simulink model "article"  (R2020a)
settings: Solver=FixedStepAuto  StartTime=0.0  StopTime=5  FixedStep=2e-4  RelTol=1e-3  AbsTol=1e-3
libraries: fl_lib x8, nesl_utility x7, ee_lib x2
settings Model: OrderedModelArguments=off  Creator=Anzin  LastModifiedBy=Anzin
settings OptimizationCC: OptimizeBlockIOStorage=off  BufferReuse=off  OptimizeDataStoreBuffers=off  BusAssignmentInplaceUpdate=off
settings DebuggingCC: SignalInfNanChecking=error  SFUnexpectedBacktrackingDiag=warning  SFNoUnconditionalDefaultTransitionDiag=warning
settings HardwareCC: ProdHWDeviceType=AMD->x86-64 (Windows64)
settings RTWCC: GenerateReport=on  BuildConfiguration=Debug  LaunchReport=on
settings CodeAppCC: ForceParamTrailComments=on  MATLABSourceComments=on  EnableCustomComments=on
settings GRTTargetCC: CombineSignalStateStructs=on  SupportVariableSizeSignals=on  MultiInstanceErrorCode=Warning

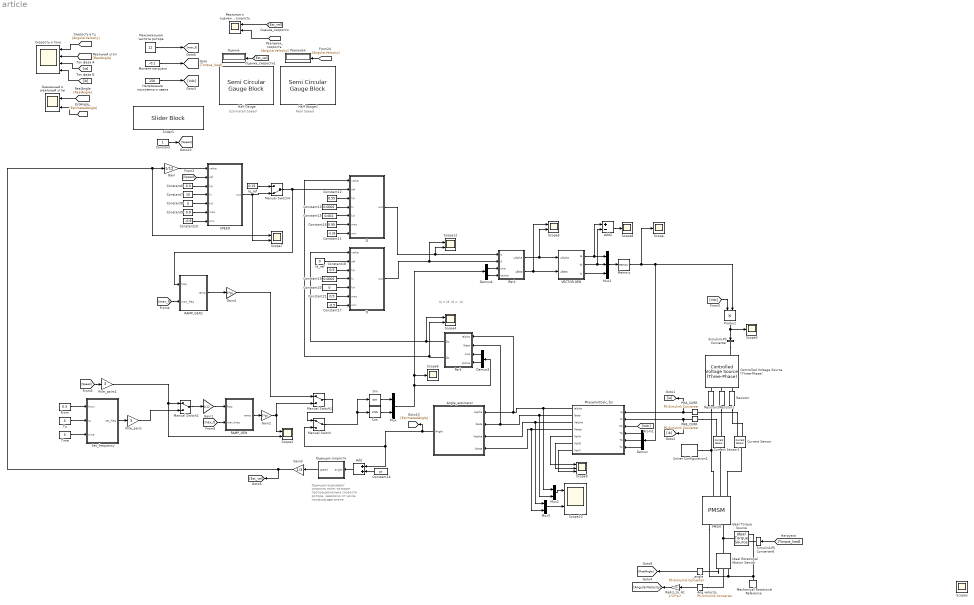
== system article ==
  note: Оценщик оценивает скорость поля, которая пропорциональна скорости ротора, зависимо от числа полюсов двигателя
  note: Real Speed
  note: Estimated Speed
  note: Iq = Id'
      | Id = -Iq'
  Add : Sum
  Add2 : Sum  Inputs=+-
  Ang velocity : nesl_utility/PS-Simulink Converter  PhysicalDomain=network_engine_domain  SubClassName=ps_output  LeftPortType=input  RightPortType=output  PseudoPeriodic=off  Frequencies=[]  Unit=inherit  AffineConversion=off
  Angle_estimator : MATLAB Function  TreatAsAtomicUnit=on
  Constant : Constant
  Constant10 : Constant  Value=-0.9
  Constant11 : Constant  Value=-0.95
  Constant12 : Constant  Value=0.55
  Constant13 : Constant  Value=0.0002
  Constant14 : Constant  Value=pi
  Constant15 : Constant  Value=0.001
  Constant16 : Constant  Value=0.95
  Constant17 : Constant  Value=-0.5
  Constant18 : Constant  Value=0.5
  Constant19 : Constant  Value=0.0002
  Constant20 : Constant  Value=0
  Constant21 : Constant  Value=0.5
  Constant6 : Constant  Value=0.3
  Constant7 : Constant  Value=10
  Constant8 : Constant  Value=0
  Constant9 : Constant  Value=0.9
  Controlled Voltage Source (Three-Phase) : ee_lib/Sources/Controlled Voltage Source (Three-Phase)
      settings: SourceProductBaseCode=PS  InternalSimscapePortConfiguration="{\"Bottom\":[],\"Left\":[{\"id\":\"S\",\"label\":\"S\",\"type\":\"input\"},{\"id\":\"n\",\"label\":\"n\",\"type\":\"foundation.electrical.electrical\"}],\"Right\":[{\"id\":\"a\",\"label\":\"a\",\"type\":\"foundation.electrical.electrical\"},{\"id\":\"b\",\"label\":\"b\",\"type\":\"foundation.electrical.electrical\"},{\"id\":\"c\",\"label\":\"c\",\"type\":\"foundation.electrical.electrical\"}],\"Top\":[]}"
  Cos : Trigonometry  Operator=cos
  Current Sensor : fl_lib/Electrical/Electrical Sensors/Current Sensor
      settings: SourceProductBaseCode=MT,SS
  Current Sensor1 : fl_lib/Electrical/Electrical Sensors/Current Sensor
      settings: SourceProductBaseCode=MT,SS
  D : MATLAB Function  TreatAsAtomicUnit=on
  Demux : Demux  Outputs=3
  Demux3 : Demux  Outputs=2
  Demux4 : Demux  Outputs=2
  From : Constant  Value=0.3
  Gain : Gain  Gain=1/12
  Gain1 : Gain  Gain=1/12
  Gain2 : Gain  Gain=2*pi
  Gain3 : Gain  Gain=1/3
  Gain4 : Gain  Gain=2*pi
  Half Gauge : SemiCircularGaugeBlock  ScaleMin=-12  ScaleMax=12
  Half Gauge1 : SemiCircularGaugeBlock  ScaleMin=-12  ScaleMax=12
  IPark : MATLAB Function  TreatAsAtomicUnit=on
  Id_ref : Constant  Value=0
  Ideal Rotational Motion Sensor : fl_lib/Mechanical/Mechanical Sensors/Ideal Rotational Motion Sensor  wrap_angle=simscape.enum.onoff.on  offset=0 rad
  Ideal Torque Source : fl_lib/Mechanical/Mechanical Sources/Ideal Torque Source
  Iq_ref : Constant  Value=0.15
  Manual Switch : ManualSwitch
  Manual Switch1 : ManualSwitch
  Manual Switch2 : ManualSwitch
  Manual Switch4 : ManualSwitch  CurrentSetting=0
  Mechanical Rotational Reference : fl_lib/Mechanical/Rotational Elements/Mechanical Rotational Reference
  Memory : Memory
  Mux : Mux  Inputs=2
  Mux1 : Mux  Inputs=3
  Mux2 : Mux  Inputs=2
  Mux3 : Mux  Inputs=2
  PHA_CURR : nesl_utility/PS-Simulink Converter  PhysicalDomain=network_engine_domain  SubClassName=ps_output  LeftPortType=input  RightPortType=output  PseudoPeriodic=off  Frequencies=[]  Unit=inherit  AffineConversion=off
  PHB_CURR : nesl_utility/PS-Simulink Converter  PhysicalDomain=network_engine_domain  SubClassName=ps_output  LeftPortType=input  RightPortType=output  PseudoPeriodic=off  Frequencies=[]  Unit=inherit  AffineConversion=off
  PMSM : ee_lib/Electromechanical/Permanent Magnet/PMSM  winding_type=ee.enum.statorconnection.wye  machine_param=ee.enum.pmsm.parameterization.constant  nPolePairs=3  pmflux_param=ee.enum.pmflux.backemfconstant  pm_flux_linkage=0.03 Wb  torque_constant=0.18 N*m/A  back_emf_constant=0.147 V/rpm  stator_param=ee.enum.statorparam.LdLqL0  Ld=10 mH  Lq=5 mH  idVec=[-200, 0, 200] A  iqVec=[-200, 0, 200] A  LdMatrix=0.0002 * ones(3, 3) H  LqMatrix=0.0002 * ones(3, 3) H  PmMatrix=0.1 * ones(3, 3) Wb  ktMatrix=0.18 * ones(3, 3) N*m/A  keMatrix=0.18 * ones(3, 3) V/(rad/s)  L0=7.5 mH  Ls=0.0002 H  Lm=-0.00002 H  Ms=0.00002 H  Rs=0.31 Ohm  zero_sequence=ee.enum.park.zerosequence.include  J=214e-4 kg*m^2  lam=0 N*m/(rad/s)  axes_param=ee.enum.rotorangle.daxis  i_d_specify=off  i_d_priority=None  i_d=0 A  i_d_nominal_specify=off  i_d_nominal_unit=A  i_d_nominal_value=1  i_q_specify=off  i_q_priority=None  i_q=0 A  i_q_nominal_specify=off  i_q_nominal_unit=A  i_q_nominal_value=1  torque_specify=off  torque_priority=None  torque=0 N*m  torque_nominal_specify=off  torque_nominal_unit=N*m  torque_nominal_value=1  angular_velocity_specify=off  angular_velocity_priority=High  angular_velocity=450 rpm  angular_velocity_nominal_specify=off  angular_velocity_nominal_unit=rpm  angular_velocity_nominal_value=1  angular_position_specify=off  angular_position_priority=High  angular_position=30 deg  angular_position_nominal_specify=off  angular_position_nominal_unit=deg  angular_position_nominal_value=1  loss_param=ee.enum.ironloss.none  losses_oc=[0, 0, 0] W  losses_sc=[0, 0, 0] W  f_losses=60 Hz  Isc_losses=95 A  Tmeas=298.15 K  alpha=3.93e-3 1/K  alpha_flux=-0.001 1/K  stator_thermal_mass=100 J/K  rotor_thermal_mass=200 J/K  Rm_percent_rotor=90  Rd_percent_rotor=30  temperatureA_specify=off  temperatureA_priority=High  temperatureA=25 degC  temperatureA_nominal_specify=off  temperatureA_nominal_unit=degC  temperatureA_nominal_value=1  temperatureB_specify=off  temperatureB_priority=High  temperatureB=25 degC  temperatureB_nominal_specify=off  temperatureB_nominal_unit=degC  temperatureB_nominal_value=1  temperatureC_specify=off  temperatureC_priority=High  temperatureC=25 degC  temperatureC_nominal_specify=off  temperatureC_nominal_unit=degC  temperatureC_nominal_value=1  temperatureR_specify=off  temperatureR_priority=High  temperatureR=25 degC  temperatureR_nominal_specify=off  temperatureR_nominal_unit=degC  temperatureR_nominal_value=1
      settings: InternalSimscapePortConfiguration="{\"Bottom\":[],\"Left\":[{\"id\":\"a\",\"label\":\"a\",\"type\":\"foundation.electrical.electrical\"},{\"id\":\"b\",\"label\":\"b\",\"type\":\"foundation.electrical.electrical\"},{\"id\":\"c\",\"label\":\"c\",\"type\":\"foundation.electrical.electrical\"},{\"id\":\"n\",\"label\":\"n\",\"type\":\"foundation.electrical.electrical\"}],\"Right\":[{\"id\":\"R\",\"label\":\"R\",\"type\":\"foundation.mechanical.rotational.rotational\"},{\"id\":\"C\",\"label\":\"C\",\"type\":\"foundation.mechanical.rotational.rotational\"}],\"Top\":[]}"
  Park : MATLAB Function  TreatAsAtomicUnit=on
  PhaseVoltCalc_fcn : MATLAB Function  TreatAsAtomicUnit=on
  Pole_pairs : Gain  Gain=3
  Pole_pairs1 : Gain  Gain=3
  Product : Product
  Q : MATLAB Function  TreatAsAtomicUnit=on
  RAMP_GEN : MATLAB Function  TreatAsAtomicUnit=on
  RAMP_GEN1 : MATLAB Function  TreatAsAtomicUnit=on
  Rad/s_to_Hz : Gain  Gain=1/(2*pi)
  Resistor : fl_lib/Electrical/Electrical Elements/Resistor  R=2 Ohm  i_specify=off  i_priority=None  i=0 A  i_nominal_specify=off  i_nominal_unit=A  i_nominal_value=1  v_specify=off  v_priority=None  v=0 V  v_nominal_specify=off  v_nominal_unit=V  v_nominal_value=1
  Resistor1 : fl_lib/Electrical/Electrical Elements/Resistor  R=2 Ohm  i_specify=off  i_priority=None  i=0 A  i_nominal_specify=off  i_nominal_unit=A  i_nominal_value=1  v_specify=off  v_priority=None  v=0 V  v_nominal_specify=off  v_nominal_unit=V  v_nominal_value=1
  Resistor2 : fl_lib/Electrical/Electrical Elements/Resistor  R=2 Ohm  i_specify=off  i_priority=None  i=0 A  i_nominal_specify=off  i_nominal_unit=A  i_nominal_value=1  v_specify=off  v_priority=None  v=0 V  v_nominal_specify=off  v_nominal_unit=V  v_nominal_value=1
  SPEED : MATLAB Function  TreatAsAtomicUnit=on
  Scope{,1,3,6,8} (5 alike) : Scope
  Scope{2,4..5,7,10,12} (6 alike) : Scope  NumInputPorts=2
  Scope9 : Scope  NumInputPorts=3
  Set_frequency : MATLAB Function  TreatAsAtomicUnit=on
  Simulink-PS Converter : nesl_utility/Simulink-PS Converter  PhysicalDomain=network_engine_domain  SubClassName=ps_input  LeftPortType=input  RightPortType=output  PseudoPeriodic=off  Frequencies=[]  NoiseDistribution=none  NoiseParameters=[]  Unit=1  AffineConversion=off  FilteringAndDerivatives=provide  SimscapeFilterOrder=1  InputFilterTimeConstant=0.001  UdotUserProvided=0
  Simulink-PS Converter6 : nesl_utility/Simulink-PS Converter  PhysicalDomain=network_engine_domain  SubClassName=ps_input  LeftPortType=input  RightPortType=output  PseudoPeriodic=off  Frequencies=[]  NoiseDistribution=none  NoiseParameters=[]  Unit=1  AffineConversion=off  FilteringAndDerivatives=provide  SimscapeFilterOrder=1  InputFilterTimeConstant=0.001  UdotUserProvided=0
  Sin : Trigonometry
  Slider1 : SliderBlock  ScaleMax=12
  Solver Configuration1 : nesl_utility/Solver Configuration  PhysicalDomain=network_engine_domain  SubClassName=solver  LeftPortType=input  RightPortType=generic  Tones=[]  Harmonics=[]  SimulateNoise=off  Profile=off  UseLocalSampling=off  EnableSwitchedLinearOptims=on  FrequencyDomain=off  UseCCode=off  RelTol=0.001  AbsTol=1e-06  MinStep=1e-09  ToWorkspace=off  RevertToSquareIcSolve=off  NumHomotopyIterations=100  PhasorMode=off  PhasorModeNumHarmonics=1  DoDC=off  ResidualTolerance=1e-09  UseLocalSolver=off  LocalSolverChoice=NE_BACKWARD_EULER_ADVANCER  LocalSolverSampleTime=0.001  DoFixedCost=off  MaxNonlinIter=3  MaxModeIter=2  LinearAlgebra=auto  EquationFormulation=NE_TIME_EF  DelaysMemoryBudget=1024  AutomaticFiltering=on  FilteringTimeConstant=0.001  PartitionStorageMethod=AS_NEEDED  PartitionMemoryBudget=1024  PartitionMethod=ROBUST
  Time : Constant  Value=5
  To : Constant  Value=5
  VECTOR GEN : MATLAB Function  TreatAsAtomicUnit=on
  _angle : nesl_utility/PS-Simulink Converter  PhysicalDomain=network_engine_domain  SubClassName=ps_output  LeftPortType=input  RightPortType=output  PseudoPeriodic=off  Frequencies=[]  Unit=inherit  AffineConversion=off
  Максимальная частота ротора : Constant  Value=12
  Момент нагрузки : Constant  Value=-0.1
  Напряжение постоянного звена : Constant  Value=150  SampleTime=-1
  Оцененный и реальный углы : Scope  NumInputPorts=2
  Оценка : Display
      settings: Decimation=3
  Оценщик скорости : MATLAB Function  TreatAsAtomicUnit=on
  Реальная : Display
      settings: Decimation=3
  Реальная и оцененная скорость : Scope  NumInputPorts=2
  Скорость и токи : Scope  NumInputPorts=4
  wires:
  Момент нагрузки/1 -> [Torque_load]
  Напряжение постоянного звена/1 -> [Vdc]
  Time/1 -> Set_frequency/3(time)
  [Torque_load] -> Simulink-PS Converter6/1
  [RealAngle] -> Скорость и токи/2
  [AngularVelocity] -> Скорость и токи/1
  [ia] -> Скорость и токи/3
  [ib] -> Скорость и токи/4
  [EstimatedAngle] -> Оцененный и реальный углы/2
  [Est_vel] -> Оценка/1
  [AngularVelocity] -> Реальная/1
  From/1 -> Set_frequency/1(from)
  To/1 -> Set_frequency/2(to)
  [Est_vel] -> Реальная и оцененная скорость/1
  [AngularVelocity] -> Реальная и оцененная скорость/2
  [Speed] -> Pole_pairs1/1
  Add/1 -> Оценщик скорости/1(angle)
  IPark/2(uBeta) -> Scope5/1, VECTOR GEN/2(uBeta)
  IPark/1(uAlpha) -> Scope5/2, VECTOR GEN/1(uAlpha)
  Constant14/1 -> Add/2
  PHA_CURR/1 -> PhaseVoltCalc_fcn/1(ia), [ia]
  Ang velocity/1 -> Rad/s_to_Hz/1
  Rad/s_to_Hz/1 -> [AngularVelocity]
  _angle/1 -> [RealAngle]
  [Vdc] -> PhaseVoltCalc_fcn/3(Vd)
  Demux/1 -> PhaseVoltCalc_fcn/4(Ta)
  Demux/2 -> PhaseVoltCalc_fcn/5(Tb)
  Demux/3 -> PhaseVoltCalc_fcn/6(Tc)
  PhaseVoltCalc_fcn/1(Ialpha) -> Mux2/1, Park/1(Ialpha), Angle_estimator/1(Ialpha)
  PhaseVoltCalc_fcn/2(Ibeta) -> Mux2/2, Park/2(Ibeta), Angle_estimator/2(Ibeta)
  PhaseVoltCalc_fcn/3(Valpha) -> Mux3/1, Angle_estimator/3(Valpha)
  PhaseVoltCalc_fcn/4(Vbeta) -> Mux3/2, Angle_estimator/4(Vbeta)
  Angle_estimator/1(Angle) -> [EstimatedAngle], Add/1, Manual Switch/2
  Manual Switch/1 -> Sin/1, Cos/1
  Cos/1 -> Mux/2
  Sin/1 -> Mux/1
  [Speed] -> SPEED/2(ref)
  Constant6/1 -> SPEED/3(kp)
  Constant7/1 -> SPEED/4(ki)
  Constant8/1 -> SPEED/5(kd)
  Constant9/1 -> SPEED/6(max)
  Constant10/1 -> SPEED/7(min)
  Оценщик скорости/1(speed) -> Gain3/1
  SPEED/1(out) -> Scope7/2, Manual Switch4/2
  Iq_ref/1 -> Manual Switch4/1
  Park/1(Ds) -> D/1(value), Scope4/1
  Constant11/1 -> Q/7(min)
  Constant16/1 -> Q/6(max)
  Constant15/1 -> Q/5(kd)
  Constant13/1 -> Q/4(ki)
  Constant12/1 -> Q/3(kp)
  Constant17/1 -> D/7(min)
  Constant21/1 -> D/6(max)
  Constant20/1 -> D/5(kd)
  Constant18/1 -> D/3(kp)
  Constant19/1 -> D/4(ki)
  Id_ref/1 -> D/2(ref)
  Park/2(Qs) -> Q/1(value), Scope4/2
  VECTOR GEN/1(ta) -> Add2/1, Mux1/1
  VECTOR GEN/2(tb) -> Add2/2, Mux1/2
  VECTOR GEN/3(tc) -> Mux1/3
  Constant/1 -> [Speed]
  Mux1/1 -> Memory/1
  Memory/1 -> Scope/1, Product/2, Demux/1
  Set_frequency/1(set_freq) -> Pole_pairs/1
  Product/1 -> Scope3/1, Simulink-PS Converter/1
  [Vdc] -> Product/1
  [RealAngle] -> Оцененный и реальный углы/1
  Gain/1 -> SPEED/1(value)
  Mux/1 -> Scope6/1, Demux4/1, Demux3/1
  Demux3/1 -> Park/3(sine)
  Demux3/2 -> Park/4(cosine)
  Demux4/1 -> IPark/3(sine)
  Demux4/2 -> IPark/4(cosine)
  Pole_pairs1/1 -> Scope2/2, Manual Switch2/1
  Pole_pairs/1 -> Manual Switch2/2
  Gain1/1 -> RAMP_GEN/1(freq)
  Manual Switch2/1 -> Gain1/1
  RAMP_GEN/1(ramp) -> Gain2/1
  Gain2/1 -> Scope2/1, Manual Switch1/2
  Add2/1 -> Scope8/1
  PhaseVoltCalc_fcn/5(VphA) -> Scope9/1
  PhaseVoltCalc_fcn/6(VphB) -> Scope9/2
  PhaseVoltCalc_fcn/7(VphC) -> Scope9/3
  Mux2/1 -> Scope10/1
  Mux3/1 -> Scope10/2
  PHB_CURR/1 -> [ib], PhaseVoltCalc_fcn/2(ib)
  Gain3/1 -> [Est_vel], Scope7/1, Gain/1
  Manual Switch4/1 -> RAMP_GEN1/1(freq), Q/2(ref)
  Q/1(out) -> Scope12/2, IPark/1(q)
  D/1(out) -> Scope12/1, IPark/2(d)
  RAMP_GEN1/1(ramp) -> Gain4/1
  Manual Switch1/1 -> Manual Switch/1
  Gain4/1 -> Manual Switch1/1
  Максимальная частота ротора/1 -> [max_f]
  [max_f] -> RAMP_GEN1/2(max_freq)
  [max_f] -> RAMP_GEN/2(max_freq)
  connections:
  PHA_CURR/LConn1 -- Current Sensor/RConn1
  PHB_CURR/LConn1 -- Current Sensor1/RConn1
  Simulink-PS Converter/RConn1 -- Controlled Voltage Source (Three-Phase)/LConn1
  Ideal Rotational Motion Sensor/LConn1 -- Ideal Torque Source/LConn1 -- PMSM/RConn1
  Mechanical Rotational Reference/LConn1 -- PMSM/RConn2 -- Ideal Rotational Motion Sensor/RConn1 -- Ideal Torque Source/RConn2
  Simulink-PS Converter6/RConn1 -- Ideal Torque Source/RConn1
  Ideal Rotational Motion Sensor/RConn3 -- _angle/LConn1
  Ang velocity/LConn1 -- Ideal Rotational Motion Sensor/RConn2
  Resistor2/LConn1 -- Controlled Voltage Source (Three-Phase)/RConn3
  Resistor1/LConn1 -- Controlled Voltage Source (Three-Phase)/RConn2
  Resistor/LConn1 -- Controlled Voltage Source (Three-Phase)/RConn1
  Resistor/RConn1 -- Current Sensor/RConn2
  Resistor1/RConn1 -- Current Sensor1/RConn2
  Resistor2/RConn1 -- PMSM/LConn3 -- Solver Configuration1/RConn1
  Current Sensor1/LConn1 -- PMSM/LConn2
  PMSM/LConn1 -- Current Sensor/LConn1

== matlab function article/RAMP_GEN1 ==
  data: freq input; ramp output; max_freq input
function ramp = Ramp(freq, max_freq)

persistent angle;
persistent prevAngle;

if isempty(angle)
    angle = 0;
end

if isempty(prevAngle)
    prevAngle = 0;
end

step = freq * max_freq * 2e-4;
angle = angle + step;

if angle >= 1
    angle = angle - 1;
end

ramp = angle;

== matlab function article/Оценщик скорости ==
  data: angle input; speed output
function speed = spdest(angle)

persistent prevAngle;
persistent prevSpeed;
persistent p_speed;
persistent counter;
persistent overall;

if isempty(overall)
    overall = 0;
end

if isempty(counter)
    counter = 0;
end

if isempty(p_speed)
    p_speed = 0;
end

if isempty(prevAngle)
    prevAngle = 0;
end

if isempty(prevSpeed)
    prevSpeed = 0;
end


if angle < prevAngle
    temp = (2 * pi) - prevAngle + angle;
else
    temp = angle - prevAngle;
end

prev_speed = 0.3 * ((temp * 5000) / 6.28) + 0.7 * (prevSpeed);
overall = overall + prev_speed;
counter = counter + 1;
prevSpeed = prev_speed;
prevAngle = angle;

if counter >= 500
    speed = overall / 500;
    p_speed = speed;
    counter = 0;
    overall = 0;
else
    speed = p_speed;
end

== matlab function article/Angle_estimator ==
  settings: updateMethod=DISCRETE
  data: Ialpha input; Angle output; Ibeta input; Valpha input; Vbeta input
function Angle = AngleEstimator(Ialpha, Ibeta, Valpha, Vbeta)

persistent prevIalpha;
persistent prevIbeta;
persistent L0;
persistent L1;
persistent angle;

if isempty(prevIalpha)
    prevIalpha = 0;
end

if isempty(prevIbeta)
    prevIbeta = 0;
end

if isempty(L0)
    L0 = (5e-3 + 10e-3) / 2;
end

if isempty(L1)
    L1 = (10e-3 - 5e-3) / 2;
end

if isempty(angle)
    angle = 0;
end

Ealpha = Valpha - 0.31 * Ialpha - (L0 + L1 * cos(2 * angle)) * (Ialpha - prevIalpha) / 2e-4;
Ebeta = Vbeta - 0.31 * Ibeta - (L0 - L1 * cos(2 * angle)) * (Ibeta - prevIbeta) / 2e-4;
prevIalpha = Ialpha;
prevIbeta = Ibeta;
Angle = atan2(-Ealpha, Ebeta);
angle = Angle;

== matlab function article/IPark ==
  data: q input; d input; uAlpha output; sine input; uBeta output; cosine input
function [uAlpha, uBeta]= IPark(q, d, sine, cosine)

%преобразование увеличивает амплитуду на 2/sqrt(3), делю обратно

% uAlpha = (d * cosine - q * sine) / (2 / sqrt(3));
% uBeta = (q * cosine + d * sine) / (2 / sqrt(3));

uAlpha = d * cosine - q * sine;
uBeta = q * cosine + d * sine;

== matlab function article/VECTOR GEN ==
  data: uAlpha input size=1; ta output size=1; uBeta input size=1; tb output size=1; tc output size=1
function [ta, tb, tc] = svgen(uAlpha, uBeta)

%здесь делают обратное преобразование кларк, но оно не такое как в книге
%калачева, если что взять оттуда и проверить
%попробовать код оттуда'

tmp1 = uBeta;
tmp2 = uBeta * 0.5 + uAlpha * (sqrt(3) / 2);
tmp3 = tmp2 - tmp1;

sector = 3;
if tmp2 > 0
    sector = sector - 1;
end

if tmp3 > 0
    sector = sector - 1;
end

if tmp1 < 0
    sector = 7 - sector;
end

if sector == 1 || sector == 4
    ta = tmp2; %значения прериодов нужно снормировать с базовым напряжением
    tb = tmp1 - tmp3;
    tc = -tmp2;
elseif sector == 2 || sector == 5
    ta = tmp3 + tmp2;
    tb = tmp1;
    tc = -tmp1;
else
    ta = tmp3;
    tb = -tmp3;
    tc = -(tmp1 + tmp2);
end

== matlab function article/SPEED ==
  settings: updateMethod=DISCRETE
  data: value input size=1; out output; ref input; kp input; ki input; kd input; max input; min input
function out  = PI(value, ref, kp, ki, kd, max, min)

persistent dT;
persistent prevIntegral;
persistent prevError;

if isempty(dT)
    dT = 2e-4;
end

if isempty(prevIntegral)
    prevIntegral = 0;
end

if isempty(prevError)
    prevError = 0;
end

error = ref - value;
%пока без предотвращения интегрального насыщения, но она тут реально нужна
integralTerm = prevIntegral + error * dT;
prevIntegral = integralTerm;

differencialTerm = (error - prevError);
prevError = error;

out_preranged = kp * error + ki * integralTerm + kd * differencialTerm;

if out_preranged < min
    out = min;
elseif out_preranged > max
    out = max;
else 
    out = out_preranged;
end

== matlab function article/PhaseVoltCalc_fcn ==
  settings: updateMethod=DISCRETE
  data: ia input; ib input; Ialpha output; Ibeta output; Vd input; Valpha output; Ta input; Tb input; Tc input; Vbeta output; VphA output; VphB output; VphC output
function [Ialpha, Ibeta, Valpha, Vbeta, VphA, VphB, VphC] = PhaseVoltCalc(ia, ib, Vd, Ta, Tb, Tc)

persistent out_of_phase;

if isempty(out_of_phase)
    out_of_phase = 0;
end

%clarke
Ialpha = ia / 80;
Ibeta = (2 * ib / 80 + ia / 80) / sqrt(3);

temp = (Vd / 150) / 3;
VphA = temp * (2 * Ta - Tb - Tc);
VphB = temp * (2 * Tb - Ta - Tc);
VphC = temp * (2 * Tc - Ta - Tb);

%здесь в системе альфа-бета получается что амплитуда в 2 делить на корень
%из 3 раз больше, чем задается
if out_of_phase == 1
    VphA = -VphA;
    VphB = -VphB;
end

Valpha = VphA;
Vbeta = ((2 * (VphB) + (VphA)) / sqrt(3));

== matlab function article/Q ==
  settings: updateMethod=DISCRETE
  data: value input size=1; out output; ref input; kp input; ki input; kd input; max input; min input
function out  = PI(value, ref, kp, ki, kd, max, min)

persistent dT;
persistent prevIntegral;
persistent prevError;

if isempty(dT)
    dT = 2e-4;
end

if isempty(prevIntegral)
    prevIntegral = 0;
end

if isempty(prevError)
    prevError = 0;
end

error = ref - value;
%пока без предотвращения интегрального насыщения, но она тут реально нужна
integralTerm = prevIntegral + error * dT;
prevIntegral = integralTerm;

differencialTerm = (error - prevError);
prevError = error;

out_preranged = kp * error + ki * integralTerm + kd * differencialTerm;

if out_preranged < min
    out = min;
elseif out_preranged > max
    out = max;
else 
    out = out_preranged;
end

== matlab function article/Park ==
  settings: updateMethod=DISCRETE
  data: Ialpha input; Ds output size=1; Ibeta input; sine input; Qs output size=1; cosine input
function [Ds, Qs] = Park(Ialpha, Ibeta, sine, cosine)

persistent prevId;
persistent prevIq;

if isempty(prevId)
    prevId = 0;
end

if isempty(prevIq)
    prevIq = 0;
end
% 
% Id = 0.4 * (Ialpha * cos(angle) + Ibeta * sin(angle)) + 0.6 * prevId;
% Iq = 0.4 * (Ibeta * cos(angle) - Ialpha * sin(angle)) + 0.6 * prevIq;
% prevId = Id;
% prevIq = Iq;

Ds = Ialpha * cosine + Ibeta * sine; 
Qs = Ibeta * cosine - Ialpha * sine;

== matlab function article/RAMP_GEN ==
  data: freq input; ramp output; max_freq input
function ramp = Ramp(freq, max_freq)

persistent angle;
persistent prevAngle;

if isempty(angle)
    angle = 0;
end

if isempty(prevAngle)
    prevAngle = 0;
end

step = freq * max_freq * 2e-4;
angle = angle + step;

if angle >= 1
    angle = angle - 1;
end

ramp = angle;

== matlab function article/Set_frequency ==
  data: set_freq output; from input; to input; time input
function set_freq = sf(from, to, time)

persistent freq;
persistent en;

if isempty(freq)
    freq = 0; 
end

if isempty(en)
    en = 1;
end

if en == 1
    step = (to - from) / (time * ((2e-4) ^ (-1)));
    freq = freq + step;
    if(abs(freq - to) <= abs(step + 0.05 * step))
        set_freq = to;
        en = 0;
    else
        set_freq = freq;
    end
else
    set_freq = to;
end

== matlab function article/D ==
  settings: updateMethod=DISCRETE
  data: value input size=1; out output; ref input; kp input; ki input; kd input; max input; min input
function out  = PI(value, ref, kp, ki, kd, max, min)

persistent dT;
persistent prevIntegral;
persistent prevError;

if isempty(dT)
    dT = 2e-4;
end

if isempty(prevIntegral)
    prevIntegral = 0;
end

if isempty(prevError)
    prevError = 0;
end

error = ref - value;
%пока без предотвращения интегрального насыщения, но она тут реально нужна
integralTerm = prevIntegral + error * dT;
prevIntegral = integralTerm;

differencialTerm = (error - prevError);
prevError = error;

out_preranged = kp * error + ki * integralTerm + kd * differencialTerm;

if out_preranged < min
    out = min;
elseif out_preranged > max
    out = max;
else 
    out = out_preranged;
end
